simulink model "irep_force_control_simu"  (Simulink 8.5)
settings: Solver=ode3  StartTime=0.0  StopTime=inf  FixedStep=dt  RelTol=1e-3
InitFcn:
  | IREP_DEPENDENCY
  | init_omni
  | init_filters
  | init_invivo
  | init_telemanipulation
  | init_parker_xyz
  | init_magnetic_tracker
  | init_loadcell
  | init_scopes
  | init_homing
  | init_force_control
  | init_xpc_invivo_simu
undefined symbols (not defined in the file): ang_vel_scale, B_simu, beta, camera_home_voltage, counter_offset, dt, dt_trakstar, E_Y, encoder_counts, epsilon_robust_inverse, gear_ratio, HomingFineEps, HomingRoughEps, HomingRoughVelocity, I1_primary, I1_secondary, I2_primary, I2_secondary, irep_parameters_left, irep_parameters_right, joystick_filter_coeffs, K_d, K_i, K_naive_inv, K_p, k_right, L1l, L1r, L2l, L2r, L_zeus, left_arm_home_voltage, left_x0_parallelogram, LeftArmHomingDirectionVector, LeftArmHomingIntGain, lin_vel_scale, LOADCELL_BIAS, LOADCELL_GAIN, max_conf_space_speed, N_joystick, N_pots, N_trakstar, OmegaMax, OmegaMin, orientation_epsilon, position_epsilon, pots_filter_coeffs, q_eps_backlash, quadrature_mode, r, right_arm_home_voltage, RightArmHomingDirectionVector, RightArmHomingIntGain, screw_pitch, statics_param, tau_compression_bias, tau_compression_gains, tau_neutral_deadband, tau_tension_bias, tau_tension_gains ... (+14)
libraries: slrtlib x38, xpcrtudplib x13, xpcobsoletelib x13, simulink x6, dspswit3 x2, dspsigops x1
(part 5 of 6)

== matlab function Trajectory Planner/Right Arm/High Level/Task Space/Desired Twist Module/Compute Twist ==
  data: p_des input double; R_des input double; MSG_Type input double; x_des output double; p_curr input double; R_curr input double; Vmax input double; Vmin input double; position_epsilon input double; lin_vel_scale input double; OmegaMax input double; OmegaMin input double; orientation_epsilon input double; ang_vel_scale input double
function x_des  = fcn(p_des,R_des,MSG_Type,p_curr,R_curr,Vmax,Vmin,position_epsilon,lin_vel_scale,OmegaMax,OmegaMin,orientation_epsilon,ang_vel_scale)
%--------------------------------------------------------------------------
% decode the message_type
% MSG_Type def
% bit0 = valid massage or not(enable or not)
% bit1 = time stamping requested or not (if should send back the local time or not)
enable = bitand(uint8(floor(MSG_Type)),1);
% position
position_error = p_des-p_curr;
M = norm(position_error);
% orientation
if (R_curr(:,1)'*R_des(:,1)+R_curr(:,2)'*R_des(:,2)+R_curr(:,3)'*R_des(:,3)-1) <= 0
    theta = 0;
else
    theta = acos(0.5 * (R_curr(:,1)'*R_des(:,1)+R_curr(:,2)'*R_des(:,2)+R_curr(:,3)'*R_des(:,3)-1));
end
%----------------------------------------------------------------------
if enable == 1
    if M < position_epsilon && theta < orientation_epsilon
        x_des = zeros(6,1);
    else
        n = position_error/M;
        r_non_unit = cross(R_curr(:,1),R_des(:,1))+cross(R_curr(:,2),R_des(:,2))+cross(R_curr(:,3),R_des(:,3));
        if sum(r_non_unit) == 0
            r = zeros(3,1);
        else
            r = r_non_unit/norm(r_non_unit);
        end
        if M > lin_vel_scale*position_epsilon
            LinVelMag = Vmax; % mm/s
        else
            LinVelMag = M*(Vmax-Vmin)/(position_epsilon*(lin_vel_scale-1)) + (lin_vel_scale*Vmin-Vmax)/(lin_vel_scale-1);
        end
        if theta > ang_vel_scale * orientation_epsilon
            AngVelMag = OmegaMax;
        else
            AngVelMag = theta*(OmegaMax-OmegaMin)/(orientation_epsilon*(ang_vel_scale-1))+ (ang_vel_scale*OmegaMin-OmegaMax)/(ang_vel_scale-1);
        end
        x_des = [LinVelMag*n
                 AngVelMag*r];
    end
else
    x_des = zeros(6,1);
end

== matlab function Trajectory Planner/Right Arm/High Level/Task Space/Direct Kinematics IREP/Direct Kinematic IREP ==
  data: b0 input double; b1 input double; p output double; psi input double; R output double; parameters input double
function [p,R]= fcn(b0,b1,psi,parameters)
    %#eml
    Y_OFFSET = parameters(1); % to be define in init file
    L1 = parameters(2);
    L2 = parameters(3);
    gripper_offset = parameters(4:6);
    % position of the stem
    b0_in_world = [0;0;b0];
    % position and orientation of snake base in world
    b1_in_b0 = [b1(1);Y_OFFSET;b1(2)];
    % R_b1_in_world = eye(3);
    % position of first end disk b1
    [p_disk1_in_b1 R_disk1_in_b1] = get_pose_of_constrained_frame(L1,L1,psi(1:2));
    % position of second end disk in disk1
    [p_disk2_in_disk1 R_disk2_in_disk1] = get_pose_of_constrained_frame(L2,L2,psi(3:4));
    % position of gripper tip in disk 2
    p_gripper_tip_in_disk2 = gripper_offset;
    Rz = RotationMatrix(180/pi * psi(5),[0;0;1]);
    %%%%%%%%%%%%%%%%%%%%%%%%%%%%%%%%%%%%%%%%%%%%%%%%%%%%%%%%%%%%%%%%%%%%%%%%%%%
    % Position and orientation of tip in world frame
    p = b0_in_world + b1_in_b0 + p_disk1_in_b1 + R_disk1_in_b1 * (p_disk2_in_disk1 + R_disk2_in_disk1 * p_gripper_tip_in_disk2);
    R = R_disk1_in_b1 * R_disk2_in_disk1 * Rz;
end

== matlab function Trajectory Planner/Left Arm/High Level/Task Space/Receive Desired Pose from MTM/Quaternion To Rotation ==
  data: quat input double; R output double
function R = fcn(quat)
%#eml
if norm(quat)==0
    quat = [1;0;0;0];
end
R = quat2rot(quat);

== matlab function Trajectory Planner/RZ/Arm selector ==
  data: right_b0_dot input double; b0dot output double; left_b0_dot input double
function b0dot = fcn(right_b0_dot,left_b0_dot)
%#eml
if sign(right_b0_dot)*sign(left_b0_dot)>=0 % if right and left arm agree on the moving direction
    if abs(right_b0_dot)>abs(left_b0_dot)
        b0dot = [right_b0_dot;0];
    else
        b0dot = [left_b0_dot;0];
    end
elseif sign(right_b0_dot)*sign(left_b0_dot)>=0 % if right and left arm not agree on the moving direction, listen to right
    b0dot = [right_b0_dot;0];
else
    b0dot = [0;0];
end

== matlab function Trajectory Planner/Right Arm/High Level/Task Space/Jxpsi Inverse IREP/Jxpsi Inverse IREP ==
  data: x_des input double; b0 input double; b1 input double; conf_space_dot output double; psi input double; parameters input double; weights input double; epsilon_in input double; max_ang_speed input double
function conf_space_dot   = fcn(x_des,b0,b1,psi,parameters,weights,epsilon_in,max_ang_speed)
%#eml
%--------------------------------------------------------------------------
Y_OFFSET = parameters(1); % to be define in init file
L1 = parameters(2);
L2 = parameters(3);
gripper_offset = parameters(4:6); 
e0 = zeros(3,1);
e1 = [1;0;0];
e3 = [0;0;1];
%--------------------------------------------------------------------------
%                        Direct Kinematics
%--------------------------------------------------------------------------
% position and orientation of snake base in world
b1_in_world = [b1(1);Y_OFFSET;b0+b1(2)];
% R_b1_in_world = eye(3);
% position of first end disk b1
[p_disk1_in_b1 R_disk1_in_b1] = get_pose_of_constrained_frame(L1,L1,psi(1:2));
% position of second end disk in disk1
[p_disk2_in_disk1 R_disk2_in_disk1] = get_pose_of_constrained_frame(L2,L2,psi(3:4));
% position of gripper tip in disk 2
p_gripper_tip_in_disk2 = gripper_offset;
Rz = RotationMatrix(180/pi * psi(5),[0;0;1]);
%%%%%%%%%%%%%%%%%%%%%%%%%%%%%%%%%%%%%%%%%%%%%%%%%%%%%%%%%%%%%%%%%%%%%%%%%%%
% Position and orientation of tip in world frame
p1_in_world = b1_in_world + p_disk1_in_b1;
p2_in_world = p1_in_world + R_disk1_in_b1 * p_disk2_in_disk1;
p_gripper_in_world = p2_in_world + R_disk1_in_b1 * R_disk2_in_disk1 * p_gripper_tip_in_disk2;
R = R_disk1_in_b1 * R_disk2_in_disk1 * Rz;
%--------------------------------------------------------------------------
%                           Jacobian
%--------------------------------------------------------------------------
% First Segment Jacobian
Jxpsi_1 = calculate_Jxpsi_s(L1,L1,psi(1),psi(2));
% Second Segment Jacobian
Jxpsi_2 = calculate_Jxpsi_s(L2,L2,psi(3),psi(4));
% Two-Segment Jacobian
% S1 = [eye(3),matcross(p1_in_world-p2_in_world)
%       zeros(3,3),eye(3)];
% S2 = [R_disk1_in_b1,matcross(p2_in_world-p_gripper_in_world)*R_disk1_in_b1
%       zeros(3,3),R_disk1_in_b1];
% IREP Jacobian
A = R_disk1_in_b1*Jxpsi_2(4:6,:);
Jv = [e3,e1,e3,Jxpsi_1(1:3,:)+matcross(p1_in_world-p_gripper_in_world)*Jxpsi_1(4:6,:),R_disk1_in_b1*Jxpsi_2(1:3,:)+matcross(p2_in_world-p_gripper_in_world)*A,e0];
Jw = [e0,e0,e0,Jxpsi_1(4:6,:),A,R(:,3)];
J = [Jv;Jw];
%--------------------------------------------------------------------------
%                       Jacobian Inverse
%--------------------------------------------------------------------------
w1 = weights(1);
w2 = weights(2);
w3 = weights(3);
w4 = weights(4);
w5 = weights(5);
w6 = weights(6);
w7 = weights(7);
w8 = weights(8);
W = diag([w1;w2;w3;w4;w5;w6;w7;w8]);
% S = [R',zeros(3,3);zeros(3,3),R'];
%--------------------------------------------------------------------------
% computer epsilon for robust inverse
if (psi(1) >= 87/180 * pi) || (psi(3) >= 87/180 * pi)
    epsilon = epsilon_in;
else
    epsilon = 0;
end
%--------------------------------------------------------------------------
% if the wrist reaches the limits I do not move.
% if (psi(5) >= pi/3-3*pi/180 && (x_des(6) > 0)) || (psi(5) <= -pi/3+3*pi/180 && (x_des(6) < 0))
% Jinv = pinv3(J,W,epsilon);
%     % redundancy resolution
%     conf_space_dot = Jinv * x_des;% + (eye(7)-Jinv*J) * qdot0;
% else
    Jinv = pinv3(J,W,epsilon);
    % redundancy resolution
    conf_space_dot = Jinv * x_des;% + (eye(7)-Jinv*J) * qdot0;
% end
%--------------------------------------------------------------------------
%                         Safe Check
%--------------------------------------------------------------------------
% snake_conf_space_dot_abs = zeros(4,1);
snake_conf_space_dot_abs = [abs(conf_space_dot(4));abs(conf_space_dot(5));abs(conf_space_dot(6));abs(conf_space_dot(7))];
if snake_conf_space_dot_abs(1) > max_ang_speed || snake_conf_space_dot_abs(2) > max_ang_speed || snake_conf_space_dot_abs(3) > max_ang_speed || snake_conf_space_dot_abs(4) > max_ang_speed
    snake_conf_space_dot_max = max(snake_conf_space_dot_abs);
    conf_space_dot(4:7) = conf_space_dot(4:7)/snake_conf_space_dot_max;
end
if psi(1) > 87/180 * pi && conf_space_dot(4) > 0
    conf_space_dot(4) = 0 + 2 *(87/180 * pi-psi(1));
elseif psi(3) > 87/180 * pi && conf_space_dot(6) > 0
    conf_space_dot(6) = 0 + 2 *(87/180 * pi-psi(3));
end
s = sum(isnan(conf_space_dot));
if s > 1
    conf_space_dot = zeros(8,1);
end
%--------------------------------------------------------------------------
%                      That's all Folks!
%--------------------------------------------------------------------------
% x_des_gripper = [R',zeros(3,3);zeros(3,3),R] * x_des;

== matlab function Trajectory Planner/Left Arm/High Level/Task Space/Direct Kinematics IREP/Direct Kinematic IREP ==
  data: b0 input double; b1 input double; p output double; psi input double; R output double; parameters input double
function [p,R]= fcn(b0,b1,psi,parameters)
    %#eml
    Y_OFFSET = parameters(1); % to be define in init file
    L1 = parameters(2);
    L2 = parameters(3);
    gripper_offset = parameters(4:6);
    % position of the stem
    b0_in_world = [0;0;b0];
    % position and orientation of snake base in world
    b1_in_b0 = [b1(1);Y_OFFSET;b1(2)];
    % R_b1_in_world = eye(3);
    % position of first end disk b1
    [p_disk1_in_b1 R_disk1_in_b1] = get_pose_of_constrained_frame(L1,L1,psi(1:2));
    % position of second end disk in disk1
    [p_disk2_in_disk1 R_disk2_in_disk1] = get_pose_of_constrained_frame(L2,L2,psi(3:4));
    % position of gripper tip in disk 2
    p_gripper_tip_in_disk2 = gripper_offset;
    Rz = RotationMatrix(180/pi * psi(5),[0;0;1]);
    %%%%%%%%%%%%%%%%%%%%%%%%%%%%%%%%%%%%%%%%%%%%%%%%%%%%%%%%%%%%%%%%%%%%%%%%%%%
    % Position and orientation of tip in world frame
    p = b0_in_world + b1_in_b0 + p_disk1_in_b1 + R_disk1_in_b1 * (p_disk2_in_disk1 + R_disk2_in_disk1 * p_gripper_tip_in_disk2);
    R = R_disk1_in_b1 * R_disk2_in_disk1 * Rz;
end

== matlab function Trajectory Planner/Right Arm/Low Level/Home Procedure/Homing Completion ==
  data: u input double; Homed output double; EPS input double
function Homed = fcn(u,EPS)
%#eml
u = abs(u);
Homed = (u<=EPS);

== matlab function Trajectory Planner/Right Arm/High Level/Inverse Istantaneous Kinematics/Snake inverse position ==
  data: psi input double; q output double
function q = fcn(psi)
%#eml
k_wrist = 1.35;
r = 2.4;
theta1 = psi(1);
delta1 = psi(2);
theta2 = psi(3);
delta2 = psi(4);
gamma = psi(5);

q1 = r*cos(delta1)*(theta1-pi/2);
q2 = r*cos(delta1+pi/2)*(theta1-pi/2);
q3 = q1 + r*cos(delta2)*(theta2-pi/2);
q4 = q2 + r*cos(delta2+pi/2)*(theta2-pi/2);
q5 = k_wrist* 3.6/2 * gamma;

q = [q1;q2;q3;q4;q5];

== matlab function Trajectory Planner/Left Arm/Low Level/Not And ==
  data: connected input double; enable output double; enable_home input double
function enable = fcn(connected,enable_home)
%#eml
FB = connected(1,1); % FB for front pot board
RB = connected(2,1); % RB for Rear pot board
% FB=0 means that the potentiometer cable is connected.
% to ensure both connceted, FB+RB=0.
if (FB+RB) == 0 && enable_home == 1
    enable = 1;
else
    enable = 0;
end

== matlab function Trajectory Planner/Left Arm/High Level/Task Space/Jxpsi Inverse IREP/Jxpsi Inverse IREP ==
  data: x_des input double; b0 input double; b1 input double; conf_space_dot output double; psi input double; parameters input double; weights input double; epsilon_in input double; max_ang_speed input double
function conf_space_dot  = fcn(x_des,b0,b1,psi,parameters,weights,epsilon_in,max_ang_speed)
%#eml
%--------------------------------------------------------------------------
Y_OFFSET = parameters(1); % to be define in init file
L1 = parameters(2);
L2 = parameters(3);
gripper_offset = parameters(4:6); 
e0 = zeros(3,1);
e1 = [1;0;0];
e3 = [0;0;1];
%--------------------------------------------------------------------------
%                        Direct Kinematics
%--------------------------------------------------------------------------
% position and orientation of snake base in world
b1_in_world = [b1(1);Y_OFFSET;b0+b1(2)];
% R_b1_in_world = eye(3);
% position of first end disk b1
[p_disk1_in_b1 R_disk1_in_b1] = get_pose_of_constrained_frame(L1,L1,psi(1:2));
% position of second end disk in disk1
[p_disk2_in_disk1 R_disk2_in_disk1] = get_pose_of_constrained_frame(L2,L2,psi(3:4));
% position of gripper tip in disk 2
p_gripper_tip_in_disk2 = gripper_offset;
Rz = RotationMatrix(180/pi * psi(5),[0;0;1]);
%%%%%%%%%%%%%%%%%%%%%%%%%%%%%%%%%%%%%%%%%%%%%%%%%%%%%%%%%%%%%%%%%%%%%%%%%%%
% Position and orientation of tip in world frame
p1_in_world = b1_in_world + p_disk1_in_b1;
p2_in_world = p1_in_world + R_disk1_in_b1 * p_disk2_in_disk1;
p_gripper_in_world = p2_in_world + R_disk1_in_b1 * R_disk2_in_disk1 * p_gripper_tip_in_disk2;
R = R_disk1_in_b1 * R_disk2_in_disk1 * Rz;
%--------------------------------------------------------------------------
%                           Jacobian
%--------------------------------------------------------------------------
% First Segment Jacobian
Jxpsi_1 = calculate_Jxpsi_s(L1,L1,psi(1),psi(2));
% Second Segment Jacobian
Jxpsi_2 = calculate_Jxpsi_s(L2,L2,psi(3),psi(4));
% Two-Segment Jacobian
% S1 = [eye(3),matcross(p1_in_world-p2_in_world)
%       zeros(3,3),eye(3)];
% S2 = [R_disk1_in_b1,matcross(p2_in_world-p_gripper_in_world)*R_disk1_in_b1
%       zeros(3,3),R_disk1_in_b1];
% IREP Jacobian
A = R_disk1_in_b1*Jxpsi_2(4:6,:);
Jv = [e3,e1,e3,Jxpsi_1(1:3,:)+matcross(p1_in_world-p_gripper_in_world)*Jxpsi_1(4:6,:),R_disk1_in_b1*Jxpsi_2(1:3,:)+matcross(p2_in_world-p_gripper_in_world)*A,e0];
Jw = [e0,e0,e0,Jxpsi_1(4:6,:),A,R(:,3)];
J = [Jv;Jw];
%--------------------------------------------------------------------------
%                       Jacobian Inverse
%--------------------------------------------------------------------------
w1 = weights(1);
w2 = weights(2);
w3 = weights(3);
w4 = weights(4);
w5 = weights(5);
w6 = weights(6);
w7 = weights(7);
w8 = weights(8);
W = diag([w1;w2;w3;w4;w5;w6;w7;w8]);
S = [R',zeros(3,3);zeros(3,3),R'];
%--------------------------------------------------------------------------
% computer epsilon for robust inverse
if (psi(1) >= 87/180 * pi) || (psi(3) >= 87/180 * pi)
    epsilon = epsilon_in;
else
    epsilon = 0;
end
%--------------------------------------------------------------------------
% if the wrist reaches the limits I do not move.
% if (psi(5) >= pi/3-3*pi/180 && (x_des(6) > 0)) || (psi(5) <= -pi/3+3*pi/180 && (x_des(6) < 0))
%     conf_space_dot = zeros(8,1);
% %     Jxpsi_in_gripper = S*J;
% %     Jxpsi_in_gripper_wave = Jxpsi_in_gripper(1:5,:);
% %     W_inv_wave = W_inv;
% %     Jinv_wave = pinv3(Jxpsi_in_gripper_wave,W,epsilon);
% %     Jinv_wave = W_inv_wave * Jxpsi_in_gripper_wave' / (Jxpsi_in_gripper_wave*W_inv_wave*Jxpsi_in_gripper_wave');
% %     x_des_in_gripper = S * x_des;
% %     conf_space_dot = Jinv_wave * x_des_in_gripper(1:5);%+ (eye(7)-Jinv_wave*Jxpsi_in_gripper_wave) * qdot0;
% else
    Jinv = pinv3(J,W,epsilon);
    % redundancy resolution
    conf_space_dot = Jinv * x_des;% + (eye(7)-Jinv*J) * qdot0;
% end
%--------------------------------------------------------------------------
%                         Safe Check
%--------------------------------------------------------------------------
% snake_conf_space_dot_abs = zeros(4,1);
snake_conf_space_dot_abs = [abs(conf_space_dot(4));abs(conf_space_dot(5));abs(conf_space_dot(6));abs(conf_space_dot(7))];
if snake_conf_space_dot_abs(1) > max_ang_speed || snake_conf_space_dot_abs(2) > max_ang_speed || snake_conf_space_dot_abs(3) > max_ang_speed || snake_conf_space_dot_abs(4) > max_ang_speed
    snake_conf_space_dot_max = max(snake_conf_space_dot_abs);
    conf_space_dot(4:7) = conf_space_dot(4:7)/snake_conf_space_dot_max;
end
if psi(1) > 87/180 * pi && conf_space_dot(4) > 0
    conf_space_dot(4) = 0 + 2 *(87/180 * pi-psi(1));
elseif psi(3) > 87/180 * pi && conf_space_dot(6) > 0
    conf_space_dot(6) = 0 + 2 *(87/180 * pi-psi(3));
end
s = sum(isnan(conf_space_dot));
if s > 1
    conf_space_dot = zeros(8,1);
end
%--------------------------------------------------------------------------
%                      That's all Folks!
%--------------------------------------------------------------------------

== matlab function Trajectory Planner/Left Arm/High Level/Task Space/right task space scope/R_to_axis_angle1 ==
  data: R input double; n_vec output double; theta output double
function [n_vec,theta] = AxisAngle(R)
%#eml
% Axis_angle(R) gives the rotation axis and the rotation angle extracted from rotation matrix R
% Note this function handles singular cases even if theta=0 or theta=180
% degrees, which cause the normal axis equation to become undefined.
% Written by N. Simaan
% Last updated 10/14/2012.

cos_theta=(trace(R)-1)/2;
sin_theta=(1/2)*sqrt((R(3,2)-R(2,3))^2 + (R(1,3)-R(3,1))^2 + (R(2,1)-R(1,2))^2);
theta=atan2(sin_theta,cos_theta);
index=0;
if abs(sin_theta)>1e-6 % before it was 1e-12, Long Wang changed it.
    n_cross=1/(2*sin_theta)*(R-R');
    n_vec=[-n_cross(2,3);n_cross(1,3);-n_cross(1,2)]; %disp('aaa');
    n_vec=n_vec/norm(n_vec);
else
    if cos_theta>0  %this means identity matrix
        n_vec=[0;0;0]; %I choose this arbitrarily to designate the special case for identity matrix
    else  %this is the case where theta is 180 degrees
        nx=sqrt((R(1,1)-cos_theta)/(1-cos_theta));
        ny=sqrt((R(2,2)-cos_theta)/(1-cos_theta));
        nz=sqrt((R(3,3)-cos_theta)/(1-cos_theta));
        
        %%% find the axis that best fits the given rotation matrix
        signs=[[1;1;1],...
               [1;-1;1],...
               [1;-1;-1],...
               [1;1;-1],...
               [-1;1;1],...
               [-1;-1;1],...
               [-1;-1;-1],...
               [-1;1;-1]];
        
        e=zeros(1,8); 
        
        for i=1:1:8
            n_candidate=signs(:,i).*[nx;ny;nz];
            Temp=rotd(n_candidate,theta*180/pi), %rotd takes its input in degrees
            e(1,i)=sum(sum((Temp-R).*(Temp-R)));
        end;    
              e,
        e_min=min(e); %the best fit    
        index=0
        for i=1:1:8  %find the index of the combination that produces the closest rotation
            if e(1,i)==e_min 
                index=i;
                break; 
            end;
        end;
        
        n_vec=signs(:,index).*[nx;ny;nz];
    end
end

== matlab function Trajectory Planner/Left Arm/High Level/Actuation Compensation/Parallelogram Backlash Compensatior/Backlash Compensator ==
  data: q_curr input double; q_dot_curr input double; epsilon output double; q2_comp_open input double; q2_comp_close input double
function epsilon   = fcn(q_curr,q_dot_curr,q2_comp_open,q2_comp_close)
%#eml
% if sign(q_dot_curr(1)) == 1
%     q2_epsilon = 0;
% elseif sign(q_dot_curr(2)) == -1
%     q2_epsilon = 0;
% else
%     q2_epsilon = epsilon_prev(1);
% end
% if sign(q_dot_curr(2)) == 1
%     q3_epsilon = 0.4;
% elseif sign(q_dot_curr(2)) == -1
%     q3_epsilon = -0.4;
% else
%     q3_epsilon = epsilon_prev(2);
% end
if q_dot_curr(1) > 0
    epsilon = [0
               0
               q2_comp_open];
elseif q_dot_curr(1) < 0
    epsilon = [0
               0
               q2_comp_close];
elseif q_curr(1) > 0
    epsilon = [0
               0
               q2_comp_open];
else
    epsilon = [0
               0
               0];
end
epsilon = [0
               0
               0];

== matlab function Trajectory Planner/Right Arm/High Level/Actuation Compensation/Parallelogram Backlash Compensatior/Backlash Compensator ==
  data: q_curr input double; q_dot_curr input double; epsilon output double; q1_comp_open input double; q1_comp_close input double; q2_comp_open input double; q2_comp_close input double
function epsilon   = fcn(q_curr,q_dot_curr,q1_comp_open,q1_comp_close,q2_comp_open,q2_comp_close)
%#eml
% if sign(q_dot_curr(1)) == 1
%     q2_epsilon = 0;
% elseif sign(q_dot_curr(2)) == -1
%     q2_epsilon = 0;
% else
%     q2_epsilon = epsilon_prev(1);
% end
% if sign(q_dot_curr(2)) == 1
%     q3_epsilon = 0.4;
% elseif sign(q_dot_curr(2)) == -1
%     q3_epsilon = -0.4;
% else
%     q3_epsilon = epsilon_prev(2);
% end
if q_dot_curr(1) > 0
   eps_2 = q1_comp_open;
elseif q_dot_curr(1) < 0
   eps_2 = q1_comp_close;
elseif q_curr(1) > 0
   eps_2 = q1_comp_open;
else
   eps_2 = 0;
end
if q_dot_curr(2) > 0
   eps_3 = q2_comp_open;
elseif q_dot_curr(1) < 0
   eps_3 = q2_comp_close;
elseif q_curr(1) > 0
   eps_3 = q2_comp_open;
else
   eps_3 = 0;
end
epsilon = [0;eps_2;eps_3];
epsilon = [0;0;0];

== matlab function Trajectory Planner/Left Arm/High Level/Inverse Istantaneous Kinematics/Snake inverse kinematics ==
  data: psi input double; q output double
function q = fcn(psi)
%#eml
k_wrist = 1.35;
r = 2.4;
theta1 = psi(1);
delta1 = psi(2);
theta2 = psi(3);
delta2 = psi(4);
gamma = psi(5);

q1 = r*cos(delta1)*(theta1-pi/2);
q2 = r*cos(delta1+pi/2)*(theta1-pi/2);
q3 = q1 + r*cos(delta2)*(theta2-pi/2);
q4 = q2 + r*cos(delta2+pi/2)*(theta2-pi/2);
q5 = k_wrist* 3.6/2 * gamma;

q = [q1;q2;q3;q4;q5];

== matlab function Trajectory Planner/Right Arm/Low Level/Not And ==
  data: connected input double; enable output double; enable_home input double
%This block ensures that the potentiometer cables are connected before 
% homing can proceed
function enable = fcn(connected,enable_home)
%#eml
FB = connected(1,1); % FB for front pot board
RB = connected(2,1); % RB for Rear pot board
% FB=0 means that the potentiometer cable is connected.
% to ensure both connceted, FB+RB=0.
if (FB+RB) == 0 && enable_home == 1
    enable = 1;
else
    enable = 0;
end

== matlab function Trajectory Planner/Right Arm/High Level/Actuation Compensation/wrist compensation ==
  data: epsilon input double; q_des input double; q_wrist output double
function q_wrist = fcn(epsilon,q_des)
%#eml

q_comm = q_des + [0;0;0;epsilon;0;0]; 
q_wrist = -q_comm(6)+q_comm(7);

end

== matlab function Trajectory Planner/Left Arm/High Level/Task Space/Compute Weigths/select weights ==
  data: b1 input double; W output double; psi input double; joint_limits input double; w_min input double; foot_switches input double
function W = fcn(b1,psi,joint_limits,w_min,foot_switches)
%#eml
% insertion stage
if foot_switches(2) == 0 && foot_switches(1) == 1
   %get_weight_insertion(q,q_min,q_max,n,w_min,w_max)
%    w1 = get_weight_insertion(b1(2),50,50+20,3,2,10);
   w1 = get_weight_insertion(b1(2),50,50+20,3,100,120); % modified by Nabil & Long, 2013/08/23
else
    w1 = 100;
end
% parallelogram
w2 = w_min(2) + get_weight_joint_limits(joint_limits(1),joint_limits(2),b1(1));
w3 = w_min(3) + get_weight_joint_limits(joint_limits(3),joint_limits(4),b1(2));
% stem
w4 = w_min(4) + get_weight_joint_limits(joint_limits(5),joint_limits(6),psi(1));
w5 = w_min(5);
w6 = w_min(6) + get_weight_joint_limits(joint_limits(7),joint_limits(8),psi(3));
w7 = w_min(7);
w8 = w_min(8);

W = [w1;w2;w3;w4;w5;w6;w7;w8];

== matlab function Trajectory Planner/Left Arm/High Level/Inverse Istantaneous Kinematics/Jaw Open/Close Module/Jaw Open/Close ==
  data: MSG_valid input double; u input double; y output double; MTM_GP_max input double; MTM_GP_min input double; q9_prev input double
function y = fcn(MSG_valid,u,MTM_GP_max,MTM_GP_min,q9_prev)
%#eml
%% as a result, the range of output should be (0,3.5)mm
if u>MTM_GP_max
    u = MTM_GP_max;
elseif u<MTM_GP_min
    u=MTM_GP_min;
else
    u=u;
end
if MSG_valid==1
    y = 3.5*(u-MTM_GP_min)/(MTM_GP_max - MTM_GP_min);
else
    y = q9_prev;
end

== matlab function Trajectory Planner/Right Arm/High Level/Actuation Compensation/Grad U2/Compute grad U ==
  data: conf_space input double; q input double; grad_U output double; L_p input double; r input double; E_Y input double; Ip input double; Is input double; theta_0 input double; beta input double
function grad_U  = fcn(conf_space,q,L_p,r,E_Y,Ip,Is,theta_0,beta)
%#eml
%--------------------------------------------------------------------------

theta = conf_space(6);
delta = conf_space(7);
q1 = q(6);
q2 = q(7);

L1 = L_p + q1;
L2 = L_p + q2;
L3 = L_p - q1;
L4 = L_p - q2;

Theta = theta - theta_0;

grad_U = E_Y*[Theta*(Ip/L_p+Is/L1+Is/L2+Is/L3+Is/L4)-0.5*Theta^2*r*Is*(cos(delta)/L1^2+cos(delta+beta)/L2^2+cos(delta+2*beta)/L3^2+cos(delta+3*beta)/L4^2);
                0.5*Theta^3*r*Is*(sin(delta)/L1^2+sin(delta+beta)/L2^2+sin(delta+2*beta)/L3^2+sin(delta+3*beta)/L4^2)];

== matlab function Trajectory Planner/Right Arm/High Level/Actuation Compensation/Compute Taus/Compute Tau ==
  data: GradU input double; conf_space input double; tau output double; k_right input double
function tau  = fcn(GradU,conf_space,k_right)
psi = conf_space(4:7);
Jqpsi1 = Jqpsi_invivo(psi(1:2),k_right(1));
Jqpsi2 = Jqpsi_invivo(psi(3:4),k_right(2));
%#eml
Jqpsi = [Jqpsi1,zeros(2,2)
         Jqpsi1,Jqpsi2];
tau = Jqpsi' \ GradU;

== matlab function Dual daVinci MTM/scopes/R_to_axis_angle1 ==
  data: R input double; n_vec output double; theta output double
function [n_vec,theta] = fcn(R)
%#eml
% Axis_angle(R) gives the rotation axis and the rotation angle extracted from rotation matrix R
% Note this function handles singular cases even if theta=0 or theta=180
% degrees, which cause the normal axis equation to become undefined.
% Written by N. Simaan
% Last updated 10/14/2012.

cos_theta=(trace(R)-1)/2;
sin_theta=(1/2)*sqrt((R(3,2)-R(2,3))^2 + (R(1,3)-R(3,1))^2 + (R(2,1)-R(1,2))^2);
theta=atan2(sin_theta,cos_theta);
index=0;
if abs(sin_theta)>1e-6 % before it was 1e-12, Long Wang changed it.
    n_cross=1/(2*sin_theta)*(R-R');
    n_vec=[-n_cross(2,3);n_cross(1,3);-n_cross(1,2)]; %disp('aaa');
    n_vec=n_vec/norm(n_vec);
else
    if cos_theta>0  %this means identity matrix
        n_vec=[0;0;0]; %I choose this arbitrarily to designate the special case for identity matrix
    else  %this is the case where theta is 180 degrees
        nx=sqrt((R(1,1)-cos_theta)/(1-cos_theta));
        ny=sqrt((R(2,2)-cos_theta)/(1-cos_theta));
        nz=sqrt((R(3,3)-cos_theta)/(1-cos_theta));
        
        %%% find the axis that best fits the given rotation matrix
        signs=[[1;1;1],...
               [1;-1;1],...
               [1;-1;-1],...
               [1;1;-1],...
               [-1;1;1],...
               [-1;-1;1],...
               [-1;-1;-1],...
               [-1;1;-1]];
        
        e=zeros(1,8); 
        
        for i=1:1:8
            n_candidate=signs(:,i).*[nx;ny;nz];
            Temp=rotd(n_candidate,theta*180/pi), %rotd takes its input in degrees
            e(1,i)=sum(sum((Temp-R).*(Temp-R)));
        end;    
              e,
        e_min=min(e); %the best fit    
        index=0
        for i=1:1:8  %find the index of the combination that produces the closest rotation
            if e(1,i)==e_min 
                index=i;
                break; 
            end;
        end;
        
        n_vec=signs(:,index).*[nx;ny;nz];
    end
end

== matlab function Trajectory Planner/Right Arm/High Level/Task Space/right task space scope/R_to_axis_angle1 ==
  data: R input double; n_vec output double; theta output double
function [n_vec,theta] = AxisAngle(R)
%#eml
% Axis_angle(R) gives the rotation axis and the rotation angle extracted from rotation matrix R
% Note this function handles singular cases even if theta=0 or theta=180
% degrees, which cause the normal axis equation to become undefined.
% Written by N. Simaan
% Last updated 10/14/2012.

cos_theta=(trace(R)-1)/2;
sin_theta=(1/2)*sqrt((R(3,2)-R(2,3))^2 + (R(1,3)-R(3,1))^2 + (R(2,1)-R(1,2))^2);
theta=atan2(sin_theta,cos_theta);
index=0;
if abs(sin_theta)>1e-6 % before it was 1e-12, Long Wang changed it.
    n_cross=1/(2*sin_theta)*(R-R');
    n_vec=[-n_cross(2,3);n_cross(1,3);-n_cross(1,2)]; %disp('aaa');
    n_vec=n_vec/norm(n_vec);
else
    if cos_theta>0  %this means identity matrix
        n_vec=[0;0;0]; %I choose this arbitrarily to designate the special case for identity matrix
    else  %this is the case where theta is 180 degrees
        nx=sqrt((R(1,1)-cos_theta)/(1-cos_theta));
        ny=sqrt((R(2,2)-cos_theta)/(1-cos_theta));
        nz=sqrt((R(3,3)-cos_theta)/(1-cos_theta));
        
        %%% find the axis that best fits the given rotation matrix
        signs=[[1;1;1],...
               [1;-1;1],...
               [1;-1;-1],...
               [1;1;-1],...
               [-1;1;1],...
               [-1;-1;1],...
               [-1;-1;-1],...
               [-1;1;-1]];
        
        e=zeros(1,8); 
        
        for i=1:1:8
            n_candidate=signs(:,i).*[nx;ny;nz];
            Temp=rotd(n_candidate,theta*180/pi), %rotd takes its input in degrees
            e(1,i)=sum(sum((Temp-R).*(Temp-R)));
        end;    
              e,
        e_min=min(e); %the best fit    
        index=0
        for i=1:1:8  %find the index of the combination that produces the closest rotation
            if e(1,i)==e_min 
                index=i;
                break; 
            end;
        end;
        
        n_vec=signs(:,index).*[nx;ny;nz];
    end
end

== matlab function Trajectory Planner/Right Arm/High Level/Inverse Istantaneous Kinematics/Jaw Open/Close Module/Jaw Open/Close ==
  data: MSG_valid input double; u input double; y output double; MTM_GP_max input double; MTM_GP_min input double; q9_prev input double
function y = fcn(MSG_valid,u,MTM_GP_max,MTM_GP_min,q9_prev)
%#eml
%% as a result, the range of output should be (0,3.5)mm
if MSG_valid==1
    y = 3.5*(u-MTM_GP_min)/(MTM_GP_max - MTM_GP_min);
else
    y = q9_prev;
end

== matlab function Tool Tracking port: 27000/compute offset ==
  data: u input double; y output double
function y = fcn(u)
%#eml
X_center = 640/2;
Y_center = 480/2;
if u(1) == 0 && u(2) == 0
    y = [0;0];
elseif abs(u(1)) > 640 || abs(u(2)) > 480
    y = [0;0];
else
    y = [u(1)-X_center
         -u(2)+Y_center];
end

== matlab function In-Vivo System/Potentiometers/Initialize Joystick/Embedded MATLAB Function ==
  data: V output double; u_curr input double; v_zero output double; t input double; u_prev input double
function [V,v_zero] = fcn(u_curr,t,u_prev)
%#eml

if t == 2 
    V = u_curr;
    v_zero = u_curr;
else
    V = u_curr - u_prev;
    v_zero = u_prev;
end

== matlab function Dual daVinci MTM/scopes/Quaternion To Rotation ==
  data: quat input double; R output double
function R = fcn(quat)
%#eml
if norm(quat)==0
    quat = [1;0;0;0];
end
R = quat2rot(quat);

== matlab function Trajectory Planner/Right Arm/High Level/Task Space/Compute Weigths/select weights ==
  data: b1 input double; W output double; psi input double; joint_limits input double; w_min input double; foot_switches input double
function W = fcn(b1,psi,joint_limits,w_min,foot_switches)
%#eml
% insertion stage
% if foot_switches(1) == 0
%     w1 = get_weight_insertion(b1(2),50,50+20,3,2,10);
% else
    w1 = 100;
% end
% parallelogram
w2 = w_min(2) + get_weight_joint_limits(joint_limits(1),joint_limits(2),b1(1));
w3 = w_min(3) + get_weight_joint_limits(joint_limits(3),joint_limits(4),b1(2));
% stem
w4 = w_min(4) + get_weight_joint_limits(joint_limits(5),joint_limits(6),psi(1));
w5 = w_min(5);
w6 = w_min(6) + get_weight_joint_limits(joint_limits(7),joint_limits(8),psi(3));
w7 = w_min(7);
w8 = w_min(8);%get_weight_joint_limits(joint_limits(9),joint_limits(10),psi(5));

% W_inv = diag([1/w1;1/w2;1/w3;1/w4;1/w5;1/w6;1/w7]);
W = [w1;w2;w3;w4;w5;w6;w7;w8];

== matlab function Dual daVinci MTM/scopes/Quaternion To Rotation1 ==
  data: quat input double; R output double
function R = fcn(quat)
%#eml
if norm(quat)==0
    quat = [1;0;0;0];
end
R = quat2rot(quat);

== matlab function Dual daVinci MTM/scopes/R_to_axis_angle2 ==
  data: R input double; n_vec output double; theta output double
function [n_vec,theta] = fcn(R)
%#eml
% Axis_angle(R) gives the rotation axis and the rotation angle extracted from rotation matrix R
% Note this function handles singular cases even if theta=0 or theta=180
% degrees, which cause the normal axis equation to become undefined.
% Written by N. Simaan
% Last updated 10/14/2012.

cos_theta=(trace(R)-1)/2;
sin_theta=(1/2)*sqrt((R(3,2)-R(2,3))^2 + (R(1,3)-R(3,1))^2 + (R(2,1)-R(1,2))^2);
theta=atan2(sin_theta,cos_theta);
index=0;
if abs(sin_theta)>1e-6 % before it was 1e-12, Long Wang changed it.
    n_cross=1/(2*sin_theta)*(R-R');
    n_vec=[-n_cross(2,3);n_cross(1,3);-n_cross(1,2)]; %disp('aaa');
    n_vec=n_vec/norm(n_vec);
else
    if cos_theta>0  %this means identity matrix
        n_vec=[0;0;0]; %I choose this arbitrarily to designate the special case for identity matrix
    else  %this is the case where theta is 180 degrees
        nx=sqrt((R(1,1)-cos_theta)/(1-cos_theta));
        ny=sqrt((R(2,2)-cos_theta)/(1-cos_theta));
        nz=sqrt((R(3,3)-cos_theta)/(1-cos_theta));
        
        %%% find the axis that best fits the given rotation matrix
        signs=[[1;1;1],...
               [1;-1;1],...
               [1;-1;-1],...
               [1;1;-1],...
               [-1;1;1],...
               [-1;-1;1],...
               [-1;-1;-1],...
               [-1;1;-1]];
        
        e=zeros(1,8); 
        
        for i=1:1:8
            n_candidate=signs(:,i).*[nx;ny;nz];
            Temp=rotd(n_candidate,theta*180/pi), %rotd takes its input in degrees
            e(1,i)=sum(sum((Temp-R).*(Temp-R)));
        end;    
              e,
        e_min=min(e); %the best fit    
        index=0
        for i=1:1:8  %find the index of the combination that produces the closest rotation
            if e(1,i)==e_min 
                index=i;
                break; 
            end;
        end;
        
        n_vec=signs(:,index).*[nx;ny;nz];
    end
end

== matlab function Trajectory Planner/Left Arm/High Level/Actuation Compensation/Compute Taus/Compute Tau ==
  data: GradU input double; conf_space input double; tau output double; k_right input double
function tau  = fcn(GradU,conf_space,k_right)
psi = conf_space(4:7);
Jqpsi1 = Jqpsi_invivo(psi(1:2),k_right(1));
Jqpsi2 = Jqpsi_invivo(psi(3:4),k_right(2));
%#eml
Jqpsi = [Jqpsi1,zeros(2,2)
         Jqpsi1,Jqpsi2];
tau = Jqpsi' \ GradU;

== matlab function Trajectory Planner/Left Arm/High Level/Actuation Compensation/Grad U1/Compute grad U ==
  data: conf_space input double; q input double; grad_U output double; L_p input double; r input double; E_Y input double; Ip input double; Is input double; theta_0 input double; beta input double
function grad_U  = fcn(conf_space,q,L_p,r,E_Y,Ip,Is,theta_0,beta)
%#eml
%--------------------------------------------------------------------------

theta = conf_space(4);
delta = conf_space(5);
q1 = q(4);
q2 = q(5);

L1 = L_p + q1;
L2 = L_p + q2;
L3 = L_p - q1;
L4 = L_p - q2;

Theta = theta - theta_0;

grad_U = E_Y*[Theta*(Ip/L_p+Is/L1+Is/L2+Is/L3+Is/L4)-0.5*Theta^2*r*Is*(cos(delta)/L1^2+cos(delta+beta)/L2^2+cos(delta+2*beta)/L3^2+cos(delta+3*beta)/L4^2);
                0.5*Theta^3*r*Is*(sin(delta)/L1^2+sin(delta+beta)/L2^2+sin(delta+2*beta)/L3^2+sin(delta+3*beta)/L4^2)];

== matlab function Trajectory Planner/Left Arm/High Level/Actuation Compensation/Grad U2/Compute grad U ==
  data: conf_space input double; q input double; grad_U output double; L_p input double; r input double; E_Y input double; Ip input double; Is input double; theta_0 input double; beta input double
function grad_U  = fcn(conf_space,q,L_p,r,E_Y,Ip,Is,theta_0,beta)
%#eml
%--------------------------------------------------------------------------

theta = conf_space(6);
delta = conf_space(7);
q1 = q(6);
q2 = q(7);

L1 = L_p + q1;
L2 = L_p + q2;
L3 = L_p - q1;
L4 = L_p - q2;

Theta = theta - theta_0;

grad_U = E_Y*[Theta*(Ip/L_p+Is/L1+Is/L2+Is/L3+Is/L4)-0.5*Theta^2*r*Is*(cos(delta)/L1^2+cos(delta+beta)/L2^2+cos(delta+2*beta)/L3^2+cos(delta+3*beta)/L4^2);
                0.5*Theta^3*r*Is*(sin(delta)/L1^2+sin(delta+beta)/L2^2+sin(delta+2*beta)/L3^2+sin(delta+3*beta)/L4^2)];

== matlab function Trajectory Planner/Right Arm/High Level/Actuation Compensation/Grad U1/Compute grad U ==
  data: conf_space input double; q input double; grad_U output double; L_p input double; r input double; E_Y input double; Ip input double; Is input double; theta_0 input double; beta input double
function grad_U  = fcn(conf_space,q,L_p,r,E_Y,Ip,Is,theta_0,beta)
%#eml
%--------------------------------------------------------------------------

theta = conf_space(4);
delta = conf_space(5);
q1 = q(4);
q2 = q(5);

L1 = L_p + q1;
L2 = L_p + q2;
L3 = L_p - q1;
L4 = L_p - q2;

Theta = theta - theta_0;

grad_U = E_Y*[Theta*(Ip/L_p+Is/L1+Is/L2+Is/L3+Is/L4)-0.5*Theta^2*r*Is*(cos(delta)/L1^2+cos(delta+beta)/L2^2+cos(delta+2*beta)/L3^2+cos(delta+3*beta)/L4^2);
                0.5*Theta^3*r*Is*(sin(delta)/L1^2+sin(delta+beta)/L2^2+sin(delta+2*beta)/L3^2+sin(delta+3*beta)/L4^2)];

== matlab function Dual daVinci MTM/Task Space Command/Right Arm - 5th Order Polynomial and Slerp/Embedded MATLAB Function ==
  data: p output double; p_des input double; p_curr input double; tf input double; tc input double; pdot output double; pdotdot output double; conf input double; confn output double; t0 input double; t0n output double; p0n output double; p0 input double; enable input double; RECORD output double
function [p,pdot,pdotdot,confn,t0n,p0n,RECORD] = fifth_order_p(p_des,p_curr,tf,tc,conf,t0,p0,enable)

n = 3;
RECORD = 0;

if enable == 0                  % Configuration space is not used (pdot = 0). 
    p = p_curr;
    pdotdot = zeros(n,1);
    pdot = zeros(n,1);          % However we do want to record the current 
    confn = 0;                  % position in order to be ready as soon 
    t0n = tc;                   % as the enable becomes 1. 
    p0n = p_curr;
else
    if (p_des-p0)'*(p_des-p0) > 0
        if conf == 0                % conf = 0 means that the 5th order poly 
            p0n = p0;               % is not configured for the desired trajectory.
            t0n = tc;               % Therefore, the block is initialized.
            confn = 1;
            pdot = zeros(n,1);
            p = p0;
            pdotdot = zeros(n,1);
        else
            p0n = p0;
            t0n = t0;
            confn = conf;
            % 5th order polynomial
            a0 = p0;
            a4 = -15*(p_des-p0);
            a3 = -2/3 * a4;
            a5 = -2/5 * a4;
            t = tc-t0;
            tau = t/tf;
            if t < tf
                RECORD = 1;
                p = a0 + a3 * tau^3 + a4 * tau^4 + a5 * tau^5;
                pdot = 3*a3*t^2/tf^3 + 4*a4*t^3/tf^4 + 5*a5*t^4/tf^5;
                pdotdot = 6*a3*t/tf^3 + 12*a4*t^2/tf^4 + 20*a5*t^3/tf^5;
            else
                p = p_des;
                pdot = zeros(n,1);
                pdotdot = zeros(n,1);
                p0n = p_des;
            end
        end
    else
        p = p_des;
        pdot = zeros(n,1);
        pdotdot = zeros(n,1);
        confn = 0;
        p0n = p0;
        t0n = t0;
    end
end
%------------------------------------------------------------------------

== matlab function In-Vivo System/Magnetic Tracker 125 Hz/process trak1/trakstar_to_pose ==
  data: u input double; sensor output double
function sensor= trak2pose(u)
%#eml
%   Frame definitions:
%   tb: the base frame of trakstar
%   n:  the norm (the X axis of trasmitter)
u = round(u*100)/100;
orig_pos = u(1:3);
n_in_tb = RotationMatrix(u(4),[0;0;1])*RotationMatrix(u(5),[0;1;0])*[1;0;0];
sensor = [orig_pos(:);n_in_tb(:)] ;

== matlab function Trajectory Planner/UDP_SendTo_MTM/Right_UDP/MSG_Decoding ==
  data: MSG_Type input double; EN output double
function EN = Decode(MSG_Type)
%#eml
% decode the message_type
% MSG_Type def
% bit0 = valid massage or not(enable or not)
% bit1 = time stamping requested or not (if should send back the local time or not)
enable = bitand(uint8(floor(MSG_Type)),2);
EN= double(enable);

== matlab function Trajectory Planner/Right Arm/High Level/Actuation Compensation/get q_dot sign/compute q_dot ==
  data: conf_space input double; conf_space_dot input double; q_dot output double
function q_dot = fcn(conf_space,conf_space_dot)
%#eml
%   q_dot is (8X1)
t1 = conf_space(4);
d1 = conf_space(5);
t2 = conf_space(6);
d2 = conf_space(7);
t1_dot = conf_space_dot(4);
d1_dot = conf_space_dot(5);
t2_dot = conf_space_dot(6);
d2_dot = conf_space_dot(7);
J_qpsi1 = Jqpsi_invivo([t1;d1],1);
J1 = [J_qpsi1;-J_qpsi1];
J_qpsi2 = Jqpsi_invivo([t2;d2],1);
J2 = [J_qpsi2;-J_qpsi2];
J_qpsi_aug = [J1,zeros(4,2);...
    J1,J2];
q_dot = J_qpsi_aug*[t1_dot;d1_dot;t2_dot;d2_dot];

== matlab function Trajectory Planner/Right Arm/High Level/Actuation Compensation/get q_dot sign/q_dot_sign ==
  data: q_dot_sign_in input double; q_dot_sign_out output double; q_dot_sign_prev input double
function q_dot_sign_out = fcn(q_dot_sign_in,q_dot_sign_prev)
%#eml
q_dot_sign_out=zeros(8,1);
for i=1:8
    if q_dot_sign_in(i)==0
        q_dot_sign_out(i)=q_dot_sign_prev(i);
    else
        q_dot_sign_out(i) = q_dot_sign_in(i);
    end
end

== matlab function In-Vivo System/Magnetic Tracker 125 Hz/process trak2/trakstar_to_pose ==
  data: u input double; sensor output double
function sensor= trak2pose(u)
%#eml
%   Frame definitions:
%   tb: the base frame of trakstar
%   n:  the norm (the X axis of trasmitter)
u = round(u*100)/100;
orig_pos = u(1:3);
n_in_tb = RotationMatrix(u(4),[0;0;1])*RotationMatrix(u(5),[0;1;0])*[1;0;0];
sensor = [orig_pos(:);n_in_tb(:)] ;

== matlab function Trajectory Planner/UDP_SendTo_MTM/Right_UDP/pose convert/Quaternion To Rotation ==
  data: quat input double; R output double
function R = fcn(quat)
%#eml
if norm(quat)==0
    quat = [1;0;0;0];
end
R = quat2rot(quat);

== matlab function In-Vivo System/Magnetic Tracker 125 Hz/process trak3/trakstar_to_pose ==
  data: u input double; sensor output double
function sensor= trak2pose(u)
%#eml
%   Frame definitions:
%   tb: the base frame of trakstar
%   n:  the norm (the X axis of trasmitter)
u = round(u*100)/100;
orig_pos = u(1:3);
n_in_tb = RotationMatrix(u(4),[0;0;1])*RotationMatrix(u(5),[0;1;0])*[1;0;0];
sensor = [orig_pos(:);n_in_tb(:)] ;

== matlab function Trajectory Planner/UDP_SendTo_MTM/Right_UDP/Embedded MATLAB Function ==
  data: R input double; R_vec output double
function R_vec = R_to_vec(R)
%#eml
%%  This func will cast a [3x3] rotation matrix to [9x1]
%%  The mapping will be column matrix, see for yourself.
R_vec = R(:);

== matlab function In-Vivo System/Magnetic Tracker 125 Hz/process trak4/trakstar_to_pose ==
  data: u input double; sensor output double
function sensor= trak2pose(u)
%#eml
%   Frame definitions:
%   tb: the base frame of trakstar
%   n:  the norm (the X axis of trasmitter)
u = round(u*100)/100;
orig_pos = u(1:3);
n_in_tb = RotationMatrix(u(4),[0;0;1])*RotationMatrix(u(5),[0;1;0])*[1;0;0];
sensor = [orig_pos(:);n_in_tb(:)] ;

== matlab function Trajectory Planner/Right Arm/Low Level/Home Procedure/Fine_Rough_Homing_Switch ==
  data: EnableFineHoming output double; error input double; dt input double; q_des output double; ERROR_eps input double; HomingVel input double; q_cur input double; HomedJoint output boolean; PrevHomedJoint input boolean
function [EnableFineHoming,q_des,HomedJoint] = fcn(error, dt,ERROR_eps,HomingVel,q_cur,PrevHomedJoint)
%#eml
%   By Long Wang, 2015/1/20
%   Input:
%       error       -> the current error in potentiometers
%       ERROR_eps   -> the tolenrace defined in potentiometers which will determine if within rough control range 
%       q_cur       -> the previous command
%       PrevHomedJoint  -> if homed detected from the previous time step
%       HomingVel       -> the joint velocity to command if the joint is rough homing mode
HomedJoint = (abs(error)<ERROR_eps);
HomedJoint = (HomedJoint|PrevHomedJoint); 
%   if the joint was detected homed previously, it will be forever seen as homed
%   to avoid noise on pots.
if sum(HomedJoint)==9
    % all joints are in rough homing control range, need to use fine homing
    q_des = q_cur; % stays the previous command
    EnableFineHoming = 1;
else
    %   not all joints are in rough homing control range
    %   the ones which are not, need to give constant velocity command
    %   And the other joints will be waiting untill all the joints are in Fine Homing mode
    EnableFineHoming = 0;
    velocity = (1-HomedJoint).*sign(error).*HomingVel; 
    q_des = q_cur + velocity*dt;
end

== matlab function Wrench Estimation/Embedded MATLAB Function ==
  data: Ws output double; W_seg1 output double; tau_curr input double; Psi input double; n_t input double; n_n input double; c_t input double; c_n input double; L input double; r input double; statics_param input double; probe_offset input double
function [Ws,W_seg1] = fcn(tau_curr,Psi,n_t,n_n,c_t,c_n,L,r,statics_param,probe_offset)
%#eml
q = in_vivo_invkin(Psi,r);
[Ws,W_seg1] = ...
    right_arm_wrench_estimation(tau_curr,...
    q,Psi,...
    n_t,n_n,...
    c_t,c_n,...
    L,r,...
    statics_param,...
    probe_offset);

== matlab function Trajectory Planner/Left Arm/Low Level/Home Procedure/Fine_Rough_Homing_Switch ==
  data: EnableFineHoming output double; error input double; dt input double; q_des output double; ERROR_eps input double; HomingVel input double; q_cur input double; HomedJoint output boolean; PrevHomedJoint input boolean
function [EnableFineHoming,q_des,HomedJoint] = fcn(error, dt,ERROR_eps,HomingVel,q_cur,PrevHomedJoint)
%#eml
%   By Long Wang, 2015/1/20
%   Input:
%       error       -> the current error in potentiometers
%       ERROR_eps   -> the tolenrace defined in potentiometers which will determine if within rough control range 
%       q_cur       -> the previous command
%       PrevHomedJoint  -> if homed detected from the previous time step
%       HomingVel       -> the joint velocity to command if the joint is rough homing mode
HomedJoint = (abs(error)<ERROR_eps);
HomedJoint = (HomedJoint|PrevHomedJoint); 
%   if the joint was detected homed previously, it will be forever seen as homed
%   to avoid noise on pots.
if sum(HomedJoint)==9
    % all joints are in rough homing control range, need to use fine homing
    q_des = q_cur; % stays the previous command
    EnableFineHoming = 1;
else
    %   not all joints are in rough homing control range
    %   the ones which are not, need to give constant velocity command
    %   And the other joints will be waiting untill all the joints are in Fine Homing mode
    EnableFineHoming = 0;
    velocity = (1-HomedJoint).*sign(error).*HomingVel; 
    q_des = q_cur + velocity*dt;
end

== matlab function Trajectory Planner/Left Arm/Low Level/Home Procedure/Homing Flags/Homing Completion ==
  data: u input double; Homed output double; EPS input double; dt input double; Homed_T output double; Homed_T_prev input double
function [Homed,Homed_T] = fcn(u,EPS,dt,Homed_T_prev)
%#eml
Homed_T = zeros(9,1);
u = abs(u);
Homed = (u<=EPS);
for i=1:9
    if Homed(i)
        Homed_T(i) = Homed_T_prev(i) + dt; %increment timer
    else
        Homed_T(i) = 0; % reset timer
    end
end
